simulink model "simulink_upp2"  (R2015b)
settings: Solver=VariableStepAuto  StartTime=0.0  StopTime=4  RelTol=1e-3
values from neighbouring files (symbols this model uses):
  P_init = eye(n+m+1)    [Matlab_uppg2.m]
  theta_init = zeros(n+m+1,1)    [Matlab_uppg2.m]    (also in Matlab_uppg3.m = zeros(2,1))
settings Model: Creator=Albin  LastModifiedBy=Albin

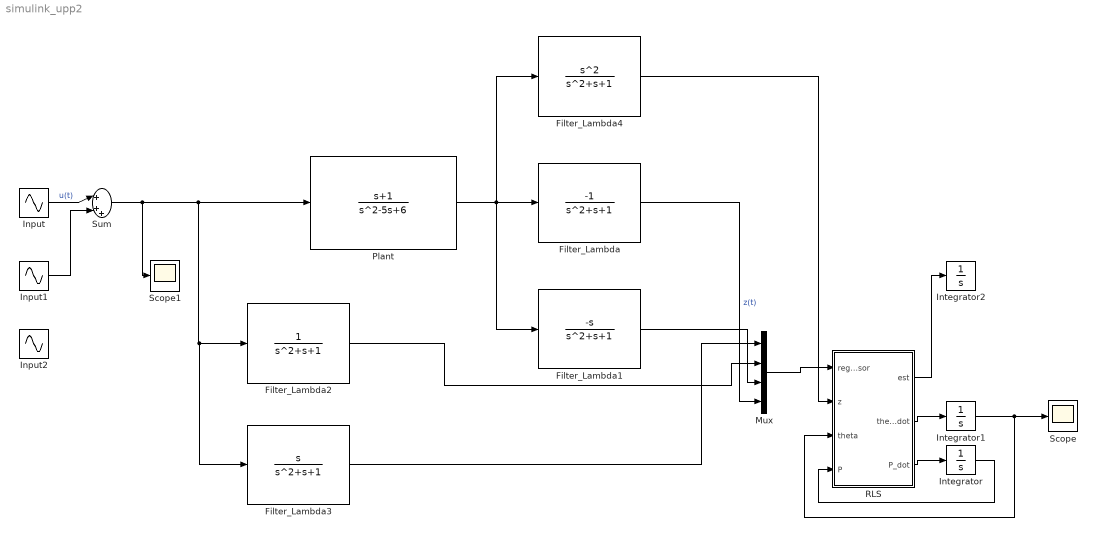
== system simulink_upp2 ==
  Filter_Lambda : TransferFcn  Numerator=[-1]  Denominator=[1 1 1]
  Filter_Lambda1 : TransferFcn  Numerator=[-1 0]  Denominator=[1 1 1]
  Filter_Lambda2 : TransferFcn  Denominator=[1 1 1]
  Filter_Lambda3 : TransferFcn  Numerator=[1 0]  Denominator=[1 1 1]
  Filter_Lambda4 : TransferFcn  Numerator=[1 0 0]  Denominator=[1 1 1]
  Input : Sin  Amplitude=4  Bias=2  SampleTime=0
  Input1 : Sin  Amplitude=4  Frequency=2  SampleTime=0
  Input2 : Sin  Bias=-2  Frequency=12.5  SampleTime=0
  Integrator : Integrator  InitialCondition=P_init
  Integrator1 : Integrator  InitialCondition=theta_init
  Integrator2 : Integrator  InitialCondition=P_init
  Mux : Mux
  Plant : TransferFcn  Numerator=[1 1]  Denominator=[1 -5 6]
  RLS : MATLAB Function  TreatAsAtomicUnit=on
  Scope : Scope
  Scope1 : Scope
  Sum : Sum  Inputs=|+++
  wires:
  Plant/1 -> Filter_Lambda4/1, Filter_Lambda1/1, Filter_Lambda/1
  Filter_Lambda/1 -> Mux/4  "z(t)"
  Filter_Lambda3/1 -> Mux/1
  Filter_Lambda2/1 -> Mux/2
  Filter_Lambda1/1 -> Mux/3
  Mux/1 -> RLS/1(regressor)
  Filter_Lambda4/1 -> RLS/2(z)
  RLS/3(P_dot) -> Integrator/1
  RLS/2(theta_dot) -> Integrator1/1
  Integrator/1 -> RLS/4(P)
  Integrator1/1 -> Scope/1, RLS/3(theta)
  RLS/1(est) -> Integrator2/1
  Input/1 -> Sum/1  "u(t)"
  Sum/1 -> Scope1/1, Filter_Lambda3/1, Filter_Lambda2/1, Plant/1
  Input1/1 -> Sum/2

== matlab function simulink_upp2/RLS ==
  data: est output; theta_dot output; regressor input; z input; P_dot output; theta input; P input
function [est,theta_dot,P_dot] = fcn(regressor,z,theta,P)
%#codegen

epsilon = z - theta'*regressor;

theta_dot = P*epsilon*regressor;
P_dot = -P*(regressor)*(regressor')*P;

est = 1/2*(z-theta'*regressor)^2;
